simulink model "switching"  (R2023b)
settings: Solver=VariableStepAuto  StartTime=0.0  StopTime=10.0  RelTol=1e-3
PreLoadFcn:
  | addpath('C:\Users\jeedu\MATLAB\Projects\final_year_project\hdlimport\switching');
libraries: hdlsllib x55
CloseFcn:
  | addpath('C:\Users\jeedu\MATLAB\Projects\final_year_project\hdlimport\switching');
  | rmpath('C:\Users\jeedu\MATLAB\Projects\final_year_project\hdlimport\switching');
settings Model: DataTypeOverride=Off  Creator=javeed  LastModifiedBy=USER
settings OptimizationCC: BlockReduction=off  ConditionallyExecuteInputs=off  DefaultParameterBehavior=Inlined  InheritOutputTypeSmallerThanSingle=on
settings DebuggingCC: ArtificialAlgebraicLoopMsg=error  InheritedTsInSrcMsg=none  SingleTaskRateTransMsg=error
settings HardwareCC: ProdBitPerPointer=32  ProdBitPerSizeT=32  ProdBitPerPtrDiffT=32  ProdLargestAtomicFloat=None  ProdIntDivRoundTo=Undefined  ProdEndianess=Unspecified  ProdWordSize=32  ProdHWDeviceType=ASIC/FPGA->ASIC/FPGA  TargetBitPerPointer=64  TargetBitPerSizeT=64  TargetBitPerPtrDiffT=64  TargetLongLongMode=on  TargetIntDivRoundTo=Zero  TargetEndianess=LittleEndian  TargetWordSize=64  TargetHWDeviceType=Custom Processor->MATLAB Host Computer  ProdEqTarget=off
settings RTWCC: GPUComputeCapability=5.0

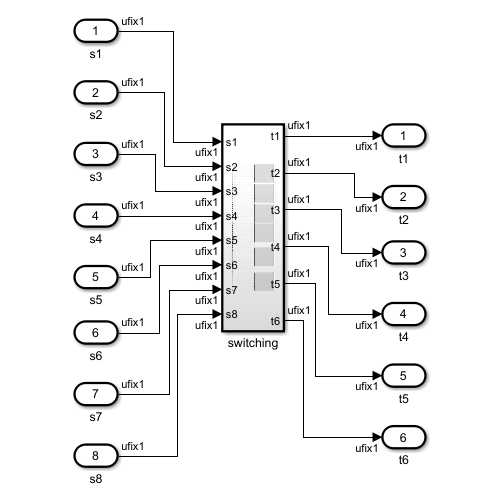
[thumbnail: Simulink's stored preview of the top-level diagram]
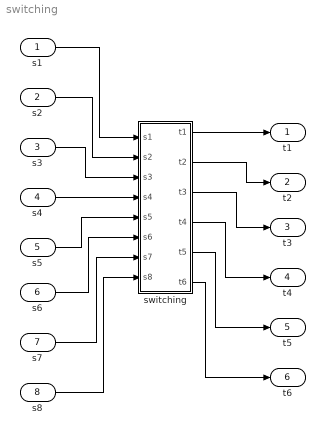
== system switching ==
  s1 : Inport  OutDataTypeStr=fixdt(0, 1, 0)  SampleTime=-1
  s2 : Inport  Port=2  OutDataTypeStr=fixdt(0, 1, 0)  SampleTime=-1
  s3 : Inport  Port=3  OutDataTypeStr=fixdt(0, 1, 0)  SampleTime=-1
  s4 : Inport  Port=4  OutDataTypeStr=fixdt(0, 1, 0)  SampleTime=-1
  s5 : Inport  Port=5  OutDataTypeStr=fixdt(0, 1, 0)  SampleTime=-1
  s6 : Inport  Port=6  OutDataTypeStr=fixdt(0, 1, 0)  SampleTime=-1
  s7 : Inport  Port=7  OutDataTypeStr=fixdt(0, 1, 0)  SampleTime=-1
  s8 : Inport  Port=8  OutDataTypeStr=fixdt(0, 1, 0)  SampleTime=-1
  switching : Subsystem
  t1 : Outport  OutDataTypeStr=fixdt(0, 1, 0)  SampleTime=-1
  t2 : Outport  Port=2  OutDataTypeStr=fixdt(0, 1, 0)  SampleTime=-1
  t3 : Outport  Port=3  OutDataTypeStr=fixdt(0, 1, 0)  SampleTime=-1
  t4 : Outport  Port=4  OutDataTypeStr=fixdt(0, 1, 0)  SampleTime=-1
  t5 : Outport  Port=5  OutDataTypeStr=fixdt(0, 1, 0)  SampleTime=-1
  t6 : Outport  Port=6  OutDataTypeStr=fixdt(0, 1, 0)  SampleTime=-1
  wires:
  s1/1 -> switching/1(s1)
  switching/5(t5) -> t5/1
  s6/1 -> switching/6(s6)
  s7/1 -> switching/7(s7)
  s2/1 -> switching/2(s2)
  s3/1 -> switching/3(s3)
  s8/1 -> switching/8(s8)
  s4/1 -> switching/4(s4)
  s5/1 -> switching/5(s5)
  switching/1(t1) -> t1/1
  switching/2(t2) -> t2/1
  switching/3(t3) -> t3/1
  switching/4(t4) -> t4/1
  switching/6(t6) -> t6/1

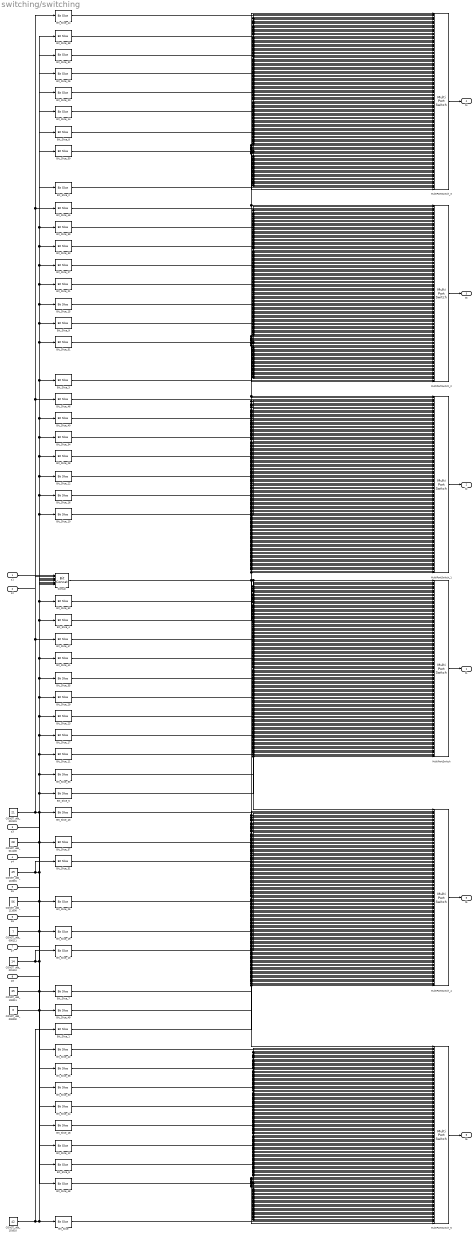
== system switching/switching ==
  s1 : Inport  OutDataTypeStr=fixdt(0, 1, 0)  SampleTime=-1
  s2 : Inport  Port=2  OutDataTypeStr=fixdt(0, 1, 0)  SampleTime=-1
  s3 : Inport  Port=3  OutDataTypeStr=fixdt(0, 1, 0)  SampleTime=-1
  s4 : Inport  Port=4  OutDataTypeStr=fixdt(0, 1, 0)  SampleTime=-1
  s5 : Inport  Port=5  OutDataTypeStr=fixdt(0, 1, 0)  SampleTime=-1
  s6 : Inport  Port=6  OutDataTypeStr=fixdt(0, 1, 0)  SampleTime=-1
  s7 : Inport  Port=7  OutDataTypeStr=fixdt(0, 1, 0)  SampleTime=-1
  s8 : Inport  Port=8  OutDataTypeStr=fixdt(0, 1, 0)  SampleTime=-1
  Bit_Slice : hdlsllib/Logic and Bit Operations/Bit Slice  lidx=double(0)  ridx=double(0)
  Bit_Slice_{1,7,13,19,25,31,37,43,49} (9 alike) : hdlsllib/Logic and Bit Operations/Bit Slice  lidx=double(1)  ridx=double(1)
  Bit_Slice_{4,10,16,22,28,34,40,46,52} (9 alike) : hdlsllib/Logic and Bit Operations/Bit Slice  lidx=double(4)  ridx=double(4)
  Bit_Slice_{5,11,17,23,29,35,41,47,53} (9 alike) : hdlsllib/Logic and Bit Operations/Bit Slice  lidx=double(5)  ridx=double(5)
  Bit_Slice_{6,12,18,24,30,36,42,48} (8 alike) : hdlsllib/Logic and Bit Operations/Bit Slice  lidx=double(0)  ridx=double(0)
  Bit_Slice_{2,8,14,20,26,32,38,44,50} (9 alike) : hdlsllib/Logic and Bit Operations/Bit Slice  lidx=double(2)  ridx=double(2)
  Bit_Slice_{3,9,15,21,27,33,39,45,51} (9 alike) : hdlsllib/Logic and Bit Operations/Bit Slice  lidx=double(3)  ridx=double(3)
  CONST_u6b_000000 : Constant  Value=0  OutDataTypeStr=fixdt(0, 6, 0)  SampleTime=-1
  CONST_u6b_000111 : Constant  Value=7  OutDataTypeStr=fixdt(0, 6, 0)  SampleTime=-1
  CONST_u6b_001110 : Constant  Value=14  OutDataTypeStr=fixdt(0, 6, 0)  SampleTime=-1
  CONST_u6b_010101 : Constant  Value=21  OutDataTypeStr=fixdt(0, 6, 0)  SampleTime=-1
  CONST_u6b_011100 : Constant  Value=28  OutDataTypeStr=fixdt(0, 6, 0)  SampleTime=-1
  CONST_u6b_100011 : Constant  Value=35  OutDataTypeStr=fixdt(0, 6, 0)  SampleTime=-1
  CONST_u6b_101010 : Constant  Value=42  OutDataTypeStr=fixdt(0, 6, 0)  SampleTime=-1
  CONST_u6b_110001 : Constant  Value=49  OutDataTypeStr=fixdt(0, 6, 0)  SampleTime=-1
  CONST_u6b_111000 : Constant  Value=56  OutDataTypeStr=fixdt(0, 6, 0)  SampleTime=-1
  Concat : hdlsllib/Logic and Bit Operations/Bit Concat  numInputs=8
  MultiPortSwitch : MultiPortSwitch  DataPortOrder=Zero-based contiguous  Inputs=130  DiagnosticForDefault=None  zeroidx=on  OutDataTypeStr=fixdt(0, 1, 0)  SampleTime=-1  SaturateOnIntegerOverflow=off  InputSameDT=off
  MultiPortSwitch_{1..5} (5 alike) : MultiPortSwitch  DataPortOrder=Zero-based contiguous  Inputs=130  DiagnosticForDefault=None  zeroidx=on  OutDataTypeStr=fixdt(0, 1, 0)  SampleTime=-1  SaturateOnIntegerOverflow=off  InputSameDT=off
  t1 : Outport  OutDataTypeStr=fixdt(0, 1, 0)  SampleTime=-1
  t2 : Outport  Port=2  OutDataTypeStr=fixdt(0, 1, 0)  SampleTime=-1
  t3 : Outport  Port=3  OutDataTypeStr=fixdt(0, 1, 0)  SampleTime=-1
  t4 : Outport  Port=4  OutDataTypeStr=fixdt(0, 1, 0)  SampleTime=-1
  t5 : Outport  Port=5  OutDataTypeStr=fixdt(0, 1, 0)  SampleTime=-1
  t6 : Outport  Port=6  OutDataTypeStr=fixdt(0, 1, 0)  SampleTime=-1
  wires:
  Bit_Slice_30/1 -> MultiPortSwitch_5/6
  Bit_Slice_25/1 -> MultiPortSwitch_4/10
  Bit_Slice_46/1 -> MultiPortSwitch_1/3
  MultiPortSwitch_2/1 -> t3/1
  Bit_Slice_43/1 -> MultiPortSwitch_4/3
  Bit_Slice_53/1 -> MultiPortSwitch/5, MultiPortSwitch/2, MultiPortSwitch/7, MultiPortSwitch/8, MultiPortSwitch/9, MultiPortSwitch/11, MultiPortSwitch/12, MultiPortSwitch/13, MultiPortSwitch/14, MultiPortSwitch/15, MultiPortSwitch/16, MultiPortSwitch/17, MultiPortSwitch/19, MultiPortSwitch/20, MultiPortSwitch/21, MultiPortSwitch/22, MultiPortSwitch/23, MultiPortSwitch/24, MultiPortSwitch/25, MultiPortSwitch/26, MultiPortSwitch/27, MultiPortSwitch/28, MultiPortSwitch/29, MultiPortSwitch/30, MultiPortSwitch/31, MultiPortSwitch/32, MultiPortSwitch/33, MultiPortSwitch/35, MultiPortSwitch/36, MultiPortSwitch/37, MultiPortSwitch/38, MultiPortSwitch/39, MultiPortSwitch/40, MultiPortSwitch/41, MultiPortSwitch/42, MultiPortSwitch/43, MultiPortSwitch/44, MultiPortSwitch/45, MultiPortSwitch/46, MultiPortSwitch/47, MultiPortSwitch/48, MultiPortSwitch/49, MultiPortSwitch/50, MultiPortSwitch/51, MultiPortSwitch/52, MultiPortSwitch/53, MultiPortSwitch/54, MultiPortSwitch/55, MultiPortSwitch/56, MultiPortSwitch/57, MultiPortSwitch/58, MultiPortSwitch/59, MultiPortSwitch/60, MultiPortSwitch/61, MultiPortSwitch/62, MultiPortSwitch/63, MultiPortSwitch/64, MultiPortSwitch/65, MultiPortSwitch/67, MultiPortSwitch/68, MultiPortSwitch/69, MultiPortSwitch/70, MultiPortSwitch/71, MultiPortSwitch/72, MultiPortSwitch/73, MultiPortSwitch/74, MultiPortSwitch/75, MultiPortSwitch/76, MultiPortSwitch/77, MultiPortSwitch/78, MultiPortSwitch/79, MultiPortSwitch/80, MultiPortSwitch/81, MultiPortSwitch/82, MultiPortSwitch/83, MultiPortSwitch/84, MultiPortSwitch/85, MultiPortSwitch/86, MultiPortSwitch/87, MultiPortSwitch/88, MultiPortSwitch/89, MultiPortSwitch/90, MultiPortSwitch/91, MultiPortSwitch/92, MultiPortSwitch/93, MultiPortSwitch/94, MultiPortSwitch/95, MultiPortSwitch/96, MultiPortSwitch/97, MultiPortSwitch/98, MultiPortSwitch/99, MultiPortSwitch/100, MultiPortSwitch/101, MultiPortSwitch/102, MultiPortSwitch/103, MultiPortSwitch/104, MultiPortSwitch/105, MultiPortSwitch/106, MultiPortSwitch/107, MultiPortSwitch/108, MultiPortSwitch/109, MultiPortSwitch/110, MultiPortSwitch/111, MultiPortSwitch/112, MultiPortSwitch/113, MultiPortSwitch/114, MultiPortSwitch/115, MultiPortSwitch/116, MultiPortSwitch/117, MultiPortSwitch/118, MultiPortSwitch/119, MultiPortSwitch/120, MultiPortSwitch/121, MultiPortSwitch/122, MultiPortSwitch/123, MultiPortSwitch/124, MultiPortSwitch/125, MultiPortSwitch/126, MultiPortSwitch/127, MultiPortSwitch/128, MultiPortSwitch/129, MultiPortSwitch/131
  Bit_Slice_44/1 -> MultiPortSwitch_3/3
  Bit_Slice_16/1 -> MultiPortSwitch_1/34
  MultiPortSwitch_5/1 -> t6/1
  Bit_Slice_10/1 -> MultiPortSwitch_1/66
  MultiPortSwitch_3/1 -> t4/1
  Bit_Slice_4/1 -> MultiPortSwitch_1/130
  Bit_Slice_38/1 -> MultiPortSwitch_3/4
  MultiPortSwitch_4/1 -> t5/1
  Bit_Slice_48/1 -> MultiPortSwitch_5/104, MultiPortSwitch_5/105, MultiPortSwitch_5/103, MultiPortSwitch_5/128, MultiPortSwitch_5/129, MultiPortSwitch_5/127, MultiPortSwitch_5/126, MultiPortSwitch_5/125, MultiPortSwitch_5/124, MultiPortSwitch_5/123, MultiPortSwitch_5/122, MultiPortSwitch_5/121, MultiPortSwitch_5/120, MultiPortSwitch_5/119, MultiPortSwitch_5/118, MultiPortSwitch_5/117, MultiPortSwitch_5/116, MultiPortSwitch_5/115, MultiPortSwitch_5/114, MultiPortSwitch_5/113, MultiPortSwitch_5/112, MultiPortSwitch_5/111, MultiPortSwitch_5/110, MultiPortSwitch_5/109, MultiPortSwitch_5/108, MultiPortSwitch_5/107, MultiPortSwitch_5/106, MultiPortSwitch_5/5, MultiPortSwitch_5/2, MultiPortSwitch_5/7, MultiPortSwitch_5/8, MultiPortSwitch_5/9, MultiPortSwitch_5/11, MultiPortSwitch_5/12, MultiPortSwitch_5/13, MultiPortSwitch_5/14, MultiPortSwitch_5/15, MultiPortSwitch_5/16, MultiPortSwitch_5/17, MultiPortSwitch_5/19, MultiPortSwitch_5/20, MultiPortSwitch_5/21, MultiPortSwitch_5/22, MultiPortSwitch_5/23, MultiPortSwitch_5/24, MultiPortSwitch_5/25, MultiPortSwitch_5/26, MultiPortSwitch_5/27, MultiPortSwitch_5/28, MultiPortSwitch_5/29, MultiPortSwitch_5/30, MultiPortSwitch_5/31, MultiPortSwitch_5/32, MultiPortSwitch_5/33, MultiPortSwitch_5/35, MultiPortSwitch_5/36, MultiPortSwitch_5/37, MultiPortSwitch_5/38, MultiPortSwitch_5/39, MultiPortSwitch_5/40, MultiPortSwitch_5/41, MultiPortSwitch_5/42, MultiPortSwitch_5/43, MultiPortSwitch_5/44, MultiPortSwitch_5/45, MultiPortSwitch_5/46, MultiPortSwitch_5/47, MultiPortSwitch_5/48, MultiPortSwitch_5/49, MultiPortSwitch_5/50, MultiPortSwitch_5/51, MultiPortSwitch_5/52, MultiPortSwitch_5/53, MultiPortSwitch_5/54, MultiPortSwitch_5/55, MultiPortSwitch_5/56, MultiPortSwitch_5/57, MultiPortSwitch_5/58, MultiPortSwitch_5/59, MultiPortSwitch_5/60, MultiPortSwitch_5/61, MultiPortSwitch_5/62, MultiPortSwitch_5/63, MultiPortSwitch_5/64, MultiPortSwitch_5/65, MultiPortSwitch_5/67, MultiPortSwitch_5/68, MultiPortSwitch_5/69, MultiPortSwitch_5/70, MultiPortSwitch_5/71, MultiPortSwitch_5/72, MultiPortSwitch_5/73, MultiPortSwitch_5/74, MultiPortSwitch_5/75, MultiPortSwitch_5/76, MultiPortSwitch_5/77, MultiPortSwitch_5/78, MultiPortSwitch_5/79, MultiPortSwitch_5/80, MultiPortSwitch_5/81, MultiPortSwitch_5/82, MultiPortSwitch_5/83, MultiPortSwitch_5/84, MultiPortSwitch_5/85, MultiPortSwitch_5/86, MultiPortSwitch_5/87, MultiPortSwitch_5/88, MultiPortSwitch_5/89, MultiPortSwitch_5/90, MultiPortSwitch_5/91, MultiPortSwitch_5/92, MultiPortSwitch_5/93, MultiPortSwitch_5/94, MultiPortSwitch_5/95, MultiPortSwitch_5/96, MultiPortSwitch_5/102, MultiPortSwitch_5/98, MultiPortSwitch_5/97, MultiPortSwitch_5/99, MultiPortSwitch_5/100, MultiPortSwitch_5/101, MultiPortSwitch_5/131
  Bit_Slice_24/1 -> MultiPortSwitch_5/10
  Bit_Slice_20/1 -> MultiPortSwitch_3/18
  Bit_Slice_42/1 -> MultiPortSwitch_5/3
  Bit_Slice_22/1 -> MultiPortSwitch_1/18
  Bit_Slice_34/1 -> MultiPortSwitch_1/6
  Bit_Slice_17/1 -> MultiPortSwitch/34
  Bit_Slice_49/1 -> MultiPortSwitch_4/2, MultiPortSwitch_4/5, MultiPortSwitch_4/7, MultiPortSwitch_4/8, MultiPortSwitch_4/9, MultiPortSwitch_4/11, MultiPortSwitch_4/12, MultiPortSwitch_4/13, MultiPortSwitch_4/14, MultiPortSwitch_4/15, MultiPortSwitch_4/16, MultiPortSwitch_4/17, MultiPortSwitch_4/19, MultiPortSwitch_4/20, MultiPortSwitch_4/21, MultiPortSwitch_4/22, MultiPortSwitch_4/23, MultiPortSwitch_4/24, MultiPortSwitch_4/25, MultiPortSwitch_4/26, MultiPortSwitch_4/27, MultiPortSwitch_4/28, MultiPortSwitch_4/29, MultiPortSwitch_4/30, MultiPortSwitch_4/31, MultiPortSwitch_4/32, MultiPortSwitch_4/33, MultiPortSwitch_4/35, MultiPortSwitch_4/36, MultiPortSwitch_4/37, MultiPortSwitch_4/38, MultiPortSwitch_4/39, MultiPortSwitch_4/40, MultiPortSwitch_4/41, MultiPortSwitch_4/42, MultiPortSwitch_4/43, MultiPortSwitch_4/44, MultiPortSwitch_4/45, MultiPortSwitch_4/46, MultiPortSwitch_4/47, MultiPortSwitch_4/48, MultiPortSwitch_4/49, MultiPortSwitch_4/50, MultiPortSwitch_4/51, MultiPortSwitch_4/52, MultiPortSwitch_4/53, MultiPortSwitch_4/54, MultiPortSwitch_4/55, MultiPortSwitch_4/56, MultiPortSwitch_4/57, MultiPortSwitch_4/58, MultiPortSwitch_4/59, MultiPortSwitch_4/60, MultiPortSwitch_4/61, MultiPortSwitch_4/62, MultiPortSwitch_4/63, MultiPortSwitch_4/64, MultiPortSwitch_4/65, MultiPortSwitch_4/67, MultiPortSwitch_4/68, MultiPortSwitch_4/69, MultiPortSwitch_4/70, MultiPortSwitch_4/71, MultiPortSwitch_4/72, MultiPortSwitch_4/73, MultiPortSwitch_4/74, MultiPortSwitch_4/75, MultiPortSwitch_4/76, MultiPortSwitch_4/77, MultiPortSwitch_4/78, MultiPortSwitch_4/79, MultiPortSwitch_4/80, MultiPortSwitch_4/81, MultiPortSwitch_4/82, MultiPortSwitch_4/83, MultiPortSwitch_4/84, MultiPortSwitch_4/85, MultiPortSwitch_4/86, MultiPortSwitch_4/87, MultiPortSwitch_4/88, MultiPortSwitch_4/89, MultiPortSwitch_4/90, MultiPortSwitch_4/91, MultiPortSwitch_4/92, MultiPortSwitch_4/93, MultiPortSwitch_4/94, MultiPortSwitch_4/95, MultiPortSwitch_4/96, MultiPortSwitch_4/97, MultiPortSwitch_4/98, MultiPortSwitch_4/99, MultiPortSwitch_4/100, MultiPortSwitch_4/101, MultiPortSwitch_4/102, MultiPortSwitch_4/103, MultiPortSwitch_4/104, MultiPortSwitch_4/105, MultiPortSwitch_4/106, MultiPortSwitch_4/107, MultiPortSwitch_4/108, MultiPortSwitch_4/109, MultiPortSwitch_4/110, MultiPortSwitch_4/111, MultiPortSwitch_4/112, MultiPortSwitch_4/113, MultiPortSwitch_4/114, MultiPortSwitch_4/115, MultiPortSwitch_4/116, MultiPortSwitch_4/117, MultiPortSwitch_4/118, MultiPortSwitch_4/119, MultiPortSwitch_4/120, MultiPortSwitch_4/121, MultiPortSwitch_4/122, MultiPortSwitch_4/123, MultiPortSwitch_4/124, MultiPortSwitch_4/125, MultiPortSwitch_4/126, MultiPortSwitch_4/127, MultiPortSwitch_4/128, MultiPortSwitch_4/129, MultiPortSwitch_4/131
  MultiPortSwitch_1/1 -> t2/1
  Bit_Slice_50/1 -> MultiPortSwitch_3/105, MultiPortSwitch_3/106, MultiPortSwitch_3/104, MultiPortSwitch_3/129, MultiPortSwitch_3/128, MultiPortSwitch_3/127, MultiPortSwitch_3/126, MultiPortSwitch_3/125, MultiPortSwitch_3/124, MultiPortSwitch_3/123, MultiPortSwitch_3/122, MultiPortSwitch_3/121, MultiPortSwitch_3/120, MultiPortSwitch_3/119, MultiPortSwitch_3/118, MultiPortSwitch_3/117, MultiPortSwitch_3/116, MultiPortSwitch_3/115, MultiPortSwitch_3/114, MultiPortSwitch_3/113, MultiPortSwitch_3/112, MultiPortSwitch_3/111, MultiPortSwitch_3/110, MultiPortSwitch_3/109, MultiPortSwitch_3/108, MultiPortSwitch_3/107, MultiPortSwitch_3/5, MultiPortSwitch_3/2, MultiPortSwitch_3/7, MultiPortSwitch_3/8, MultiPortSwitch_3/9, MultiPortSwitch_3/11, MultiPortSwitch_3/12, MultiPortSwitch_3/13, MultiPortSwitch_3/14, MultiPortSwitch_3/15, MultiPortSwitch_3/16, MultiPortSwitch_3/17, MultiPortSwitch_3/19, MultiPortSwitch_3/20, MultiPortSwitch_3/21, MultiPortSwitch_3/22, MultiPortSwitch_3/23, MultiPortSwitch_3/24, MultiPortSwitch_3/25, MultiPortSwitch_3/26, MultiPortSwitch_3/27, MultiPortSwitch_3/28, MultiPortSwitch_3/29, MultiPortSwitch_3/30, MultiPortSwitch_3/31, MultiPortSwitch_3/32, MultiPortSwitch_3/33, MultiPortSwitch_3/35, MultiPortSwitch_3/36, MultiPortSwitch_3/37, MultiPortSwitch_3/38, MultiPortSwitch_3/39, MultiPortSwitch_3/40, MultiPortSwitch_3/41, MultiPortSwitch_3/42, MultiPortSwitch_3/43, MultiPortSwitch_3/44, MultiPortSwitch_3/45, MultiPortSwitch_3/46, MultiPortSwitch_3/47, MultiPortSwitch_3/48, MultiPortSwitch_3/49, MultiPortSwitch_3/50, MultiPortSwitch_3/51, MultiPortSwitch_3/52, MultiPortSwitch_3/53, MultiPortSwitch_3/54, MultiPortSwitch_3/55, MultiPortSwitch_3/56, MultiPortSwitch_3/57, MultiPortSwitch_3/58, MultiPortSwitch_3/59, MultiPortSwitch_3/60, MultiPortSwitch_3/61, MultiPortSwitch_3/62, MultiPortSwitch_3/63, MultiPortSwitch_3/64, MultiPortSwitch_3/65, MultiPortSwitch_3/67, MultiPortSwitch_3/68, MultiPortSwitch_3/69, MultiPortSwitch_3/70, MultiPortSwitch_3/71, MultiPortSwitch_3/72, MultiPortSwitch_3/73, MultiPortSwitch_3/74, MultiPortSwitch_3/75, MultiPortSwitch_3/76, MultiPortSwitch_3/77, MultiPortSwitch_3/78, MultiPortSwitch_3/79, MultiPortSwitch_3/80, MultiPortSwitch_3/81, MultiPortSwitch_3/82, MultiPortSwitch_3/83, MultiPortSwitch_3/84, MultiPortSwitch_3/85, MultiPortSwitch_3/86, MultiPortSwitch_3/87, MultiPortSwitch_3/88, MultiPortSwitch_3/89, MultiPortSwitch_3/90, MultiPortSwitch_3/91, MultiPortSwitch_3/92, MultiPortSwitch_3/93, MultiPortSwitch_3/94, MultiPortSwitch_3/95, MultiPortSwitch_3/96, MultiPortSwitch_3/97, MultiPortSwitch_3/103, MultiPortSwitch_3/99, MultiPortSwitch_3/98, MultiPortSwitch_3/100, MultiPortSwitch_3/101, MultiPortSwitch_3/102, MultiPortSwitch_3/131
  MultiPortSwitch/1 -> t1/1
  Bit_Slice_51/1 -> MultiPortSwitch_2/105, MultiPortSwitch_2/104, MultiPortSwitch_2/103, MultiPortSwitch_2/129, MultiPortSwitch_2/128, MultiPortSwitch_2/127, MultiPortSwitch_2/126, MultiPortSwitch_2/125, MultiPortSwitch_2/124, MultiPortSwitch_2/123, MultiPortSwitch_2/122, MultiPortSwitch_2/121, MultiPortSwitch_2/120, MultiPortSwitch_2/119, MultiPortSwitch_2/118, MultiPortSwitch_2/117, MultiPortSwitch_2/116, MultiPortSwitch_2/115, MultiPortSwitch_2/114, MultiPortSwitch_2/113, MultiPortSwitch_2/112, MultiPortSwitch_2/111, MultiPortSwitch_2/110, MultiPortSwitch_2/109, MultiPortSwitch_2/108, MultiPortSwitch_2/107, MultiPortSwitch_2/106, MultiPortSwitch_2/5, MultiPortSwitch_2/2, MultiPortSwitch_2/7, MultiPortSwitch_2/8, MultiPortSwitch_2/9, MultiPortSwitch_2/11, MultiPortSwitch_2/12, MultiPortSwitch_2/13, MultiPortSwitch_2/14, MultiPortSwitch_2/15, MultiPortSwitch_2/16, MultiPortSwitch_2/17, MultiPortSwitch_2/19, MultiPortSwitch_2/20, MultiPortSwitch_2/21, MultiPortSwitch_2/22, MultiPortSwitch_2/23, MultiPortSwitch_2/24, MultiPortSwitch_2/25, MultiPortSwitch_2/26, MultiPortSwitch_2/27, MultiPortSwitch_2/28, MultiPortSwitch_2/29, MultiPortSwitch_2/30, MultiPortSwitch_2/31, MultiPortSwitch_2/32, MultiPortSwitch_2/33, MultiPortSwitch_2/35, MultiPortSwitch_2/36, MultiPortSwitch_2/37, MultiPortSwitch_2/38, MultiPortSwitch_2/39, MultiPortSwitch_2/40, MultiPortSwitch_2/41, MultiPortSwitch_2/42, MultiPortSwitch_2/43, MultiPortSwitch_2/44, MultiPortSwitch_2/45, MultiPortSwitch_2/46, MultiPortSwitch_2/47, MultiPortSwitch_2/48, MultiPortSwitch_2/49, MultiPortSwitch_2/50, MultiPortSwitch_2/51, MultiPortSwitch_2/52, MultiPortSwitch_2/53, MultiPortSwitch_2/54, MultiPortSwitch_2/55, MultiPortSwitch_2/56, MultiPortSwitch_2/57, MultiPortSwitch_2/58, MultiPortSwitch_2/59, MultiPortSwitch_2/60, MultiPortSwitch_2/61, MultiPortSwitch_2/62, MultiPortSwitch_2/63, MultiPortSwitch_2/64, MultiPortSwitch_2/65, MultiPortSwitch_2/67, MultiPortSwitch_2/68, MultiPortSwitch_2/69, MultiPortSwitch_2/70, MultiPortSwitch_2/71, MultiPortSwitch_2/72, MultiPortSwitch_2/73, MultiPortSwitch_2/74, MultiPortSwitch_2/75, MultiPortSwitch_2/76, MultiPortSwitch_2/77, MultiPortSwitch_2/78, MultiPortSwitch_2/79, MultiPortSwitch_2/80, MultiPortSwitch_2/81, MultiPortSwitch_2/82, MultiPortSwitch_2/83, MultiPortSwitch_2/84, MultiPortSwitch_2/85, MultiPortSwitch_2/86, MultiPortSwitch_2/87, MultiPortSwitch_2/88, MultiPortSwitch_2/89, MultiPortSwitch_2/90, MultiPortSwitch_2/91, MultiPortSwitch_2/92, MultiPortSwitch_2/93, MultiPortSwitch_2/94, MultiPortSwitch_2/95, MultiPortSwitch_2/96, MultiPortSwitch_2/102, MultiPortSwitch_2/97, MultiPortSwitch_2/98, MultiPortSwitch_2/99, MultiPortSwitch_2/100, MultiPortSwitch_2/101, MultiPortSwitch_2/131
  Bit_Slice_40/1 -> MultiPortSwitch_1/4
  Bit_Slice_23/1 -> MultiPortSwitch/18
  Bit_Slice_12/1 -> MultiPortSwitch_5/34
  s7/1 -> Concat/7
  Bit_Slice_47/1 -> MultiPortSwitch/3
  Bit_Slice_29/1 -> MultiPortSwitch/10
  Bit_Slice_45/1 -> MultiPortSwitch_2/3
  CONST_u6b_101010/1 -> Bit_Slice_3/1, Bit_Slice_2/1, Bit_Slice_4/1, Bit_Slice_5/1, Bit_Slice/1, Bit_Slice_1/1
  Bit_Slice_36/1 -> MultiPortSwitch_5/4
  Bit_Slice_32/1 -> MultiPortSwitch_3/6
  CONST_u6b_000000/1 -> Bit_Slice_51/1, Bit_Slice_50/1, Bit_Slice_52/1, Bit_Slice_53/1, Bit_Slice_48/1, Bit_Slice_49/1
  CONST_u6b_110001/1 -> Bit_Slice_33/1, Bit_Slice_32/1, Bit_Slice_34/1, Bit_Slice_35/1, Bit_Slice_30/1, Bit_Slice_31/1
  CONST_u6b_111000/1 -> Bit_Slice_27/1, Bit_Slice_26/1, Bit_Slice_28/1, Bit_Slice_29/1, Bit_Slice_24/1, Bit_Slice_25/1
  Bit_Slice_37/1 -> MultiPortSwitch_4/4
  Bit_Slice_39/1 -> MultiPortSwitch_2/4
  s2/1 -> Concat/2
  Bit_Slice_18/1 -> MultiPortSwitch_5/18
  Bit_Slice_26/1 -> MultiPortSwitch_3/10
  Bit_Slice_35/1 -> MultiPortSwitch/6
  s8/1 -> Concat/8
  Bit_Slice_41/1 -> MultiPortSwitch/4
  Bit_Slice_52/1 -> MultiPortSwitch_1/5, MultiPortSwitch_1/2, MultiPortSwitch_1/7, MultiPortSwitch_1/8, MultiPortSwitch_1/9, MultiPortSwitch_1/11, MultiPortSwitch_1/12, MultiPortSwitch_1/13, MultiPortSwitch_1/14, MultiPortSwitch_1/15, MultiPortSwitch_1/16, MultiPortSwitch_1/17, MultiPortSwitch_1/19, MultiPortSwitch_1/20, MultiPortSwitch_1/21, MultiPortSwitch_1/22, MultiPortSwitch_1/23, MultiPortSwitch_1/24, MultiPortSwitch_1/25, MultiPortSwitch_1/26, MultiPortSwitch_1/27, MultiPortSwitch_1/28, MultiPortSwitch_1/29, MultiPortSwitch_1/30, MultiPortSwitch_1/31, MultiPortSwitch_1/32, MultiPortSwitch_1/33, MultiPortSwitch_1/35, MultiPortSwitch_1/36, MultiPortSwitch_1/37, MultiPortSwitch_1/38, MultiPortSwitch_1/39, MultiPortSwitch_1/40, MultiPortSwitch_1/41, MultiPortSwitch_1/42, MultiPortSwitch_1/43, MultiPortSwitch_1/44, MultiPortSwitch_1/45, MultiPortSwitch_1/46, MultiPortSwitch_1/47, MultiPortSwitch_1/48, MultiPortSwitch_1/49, MultiPortSwitch_1/50, MultiPortSwitch_1/51, MultiPortSwitch_1/52, MultiPortSwitch_1/53, MultiPortSwitch_1/54, MultiPortSwitch_1/55, MultiPortSwitch_1/56, MultiPortSwitch_1/57, MultiPortSwitch_1/58, MultiPortSwitch_1/59, MultiPortSwitch_1/60, MultiPortSwitch_1/61, MultiPortSwitch_1/62, MultiPortSwitch_1/63, MultiPortSwitch_1/64, MultiPortSwitch_1/65, MultiPortSwitch_1/67, MultiPortSwitch_1/68, MultiPortSwitch_1/69, MultiPortSwitch_1/70, MultiPortSwitch_1/71, MultiPortSwitch_1/72, MultiPortSwitch_1/73, MultiPortSwitch_1/74, MultiPortSwitch_1/75, MultiPortSwitch_1/76, MultiPortSwitch_1/77, MultiPortSwitch_1/78, MultiPortSwitch_1/79, MultiPortSwitch_1/80, MultiPortSwitch_1/81, MultiPortSwitch_1/82, MultiPortSwitch_1/83, MultiPortSwitch_1/84, MultiPortSwitch_1/85, MultiPortSwitch_1/86, MultiPortSwitch_1/87, MultiPortSwitch_1/88, MultiPortSwitch_1/89, MultiPortSwitch_1/90, MultiPortSwitch_1/91, MultiPortSwitch_1/92, MultiPortSwitch_1/93, MultiPortSwitch_1/94, MultiPortSwitch_1/95, MultiPortSwitch_1/96, MultiPortSwitch_1/97, MultiPortSwitch_1/98, MultiPortSwitch_1/99, MultiPortSwitch_1/100, MultiPortSwitch_1/101, MultiPortSwitch_1/102, MultiPortSwitch_1/103, MultiPortSwitch_1/104, MultiPortSwitch_1/105, MultiPortSwitch_1/106, MultiPortSwitch_1/107, MultiPortSwitch_1/108, MultiPortSwitch_1/109, MultiPortSwitch_1/110, MultiPortSwitch_1/111, MultiPortSwitch_1/112, MultiPortSwitch_1/113, MultiPortSwitch_1/114, MultiPortSwitch_1/115, MultiPortSwitch_1/116, MultiPortSwitch_1/117, MultiPortSwitch_1/118, MultiPortSwitch_1/119, MultiPortSwitch_1/120, MultiPortSwitch_1/121, MultiPortSwitch_1/122, MultiPortSwitch_1/123, MultiPortSwitch_1/124, MultiPortSwitch_1/125, MultiPortSwitch_1/126, MultiPortSwitch_1/127, MultiPortSwitch_1/128, MultiPortSwitch_1/129, MultiPortSwitch_1/131
  Bit_Slice_33/1 -> MultiPortSwitch_2/6
  s5/1 -> Concat/5
  Bit_Slice_31/1 -> MultiPortSwitch_4/6
  Bit_Slice_13/1 -> MultiPortSwitch_4/34
  Bit_Slice_1/1 -> MultiPortSwitch_4/130
  s6/1 -> Concat/6
  Bit_Slice_27/1 -> MultiPortSwitch_2/10
  Bit_Slice_21/1 -> MultiPortSwitch_2/18
  Bit_Slice_28/1 -> MultiPortSwitch_1/10
  Bit_Slice_19/1 -> MultiPortSwitch_4/18
  Bit_Slice_3/1 -> MultiPortSwitch_2/130
  Bit_Slice_14/1 -> MultiPortSwitch_3/34
  Bit_Slice_15/1 -> MultiPortSwitch_2/34
  Bit_Slice_8/1 -> MultiPortSwitch_3/66
  Bit_Slice_6/1 -> MultiPortSwitch_5/66
  Bit_Slice_7/1 -> MultiPortSwitch_4/66
  Bit_Slice_9/1 -> MultiPortSwitch_2/66
  Bit_Slice_11/1 -> MultiPortSwitch/66
  Bit_Slice/1 -> MultiPortSwitch_5/130
  CONST_u6b_001110/1 -> Bit_Slice_14/1, Bit_Slice_15/1, Bit_Slice_16/1, Bit_Slice_17/1, Bit_Slice_12/1, Bit_Slice_13/1
  Bit_Slice_2/1 -> MultiPortSwitch_3/130
  Bit_Slice_5/1 -> MultiPortSwitch/130
  s4/1 -> Concat/4
  s3/1 -> Concat/3
  s1/1 -> Concat/1
  Concat/1 -> MultiPortSwitch_4/1, MultiPortSwitch/1, MultiPortSwitch_2/1, MultiPortSwitch_3/1, MultiPortSwitch_1/1, MultiPortSwitch_5/1
  CONST_u6b_100011/1 -> Bit_Slice_9/1, Bit_Slice_8/1, Bit_Slice_10/1, Bit_Slice_11/1, Bit_Slice_7/1, Bit_Slice_6/1
  CONST_u6b_011100/1 -> Bit_Slice_38/1, Bit_Slice_39/1, Bit_Slice_40/1, Bit_Slice_41/1, Bit_Slice_36/1, Bit_Slice_37/1
  CONST_u6b_000111/1 -> Bit_Slice_20/1, Bit_Slice_21/1, Bit_Slice_22/1, Bit_Slice_23/1, Bit_Slice_18/1, Bit_Slice_19/1
  CONST_u6b_010101/1 -> Bit_Slice_43/1, Bit_Slice_42/1, Bit_Slice_45/1, Bit_Slice_44/1, Bit_Slice_46/1, Bit_Slice_47/1
